simulink model "E5"  (Simulink 10.0)
settings: Solver=ode45  StartTime=0.0  StopTime=10.0  RelTol=1e-3  EnableMultiTasking=on
settings Model: Creator=tjohnson  LastModifiedBy=unknown
settings DataIOCC: LimitDataPoints=on
settings DebuggingCC: UnderspecifiedInitializationDetection=Simplified  MergeDetectMultiDrivingBlocksExec=error
settings GRTTargetCC: GeneratePreprocessorConditionals=Disable all  CombineOutputUpdateFcns=on  GRTInterface=off
settings ConfigComp: CovExternalEMLEnable=off

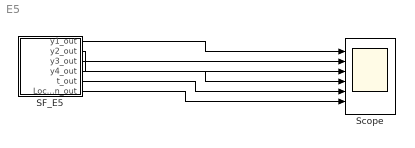
== system E5 ==
  SF_E5 : Stateflow chart  TreatAsAtomicUnit=on
  Scope : Scope  NumInputPorts=6
  wires:
  SF_E5/1(y1_out) -> Scope/1
  SF_E5/2(y2_out) -> Scope/2
  SF_E5/3(y3_out) -> Scope/3
  SF_E5/4(y4_out) -> Scope/4
  SF_E5/5(t_out) -> Scope/5
  SF_E5/6(Location_out) -> Scope/6

== stateflow chart SF_E5 ==
  settings: updateMethod=CONTINUOUS
  state E5
    du:
    y1_dot = -A * y1 - B * y1 * y3;
    y2_dot = A * y1 - M * C * y2 * y3;
    y3_dot = A * y1 - B * y1 * y3 - M * C * y2 * y3 + C * y4;
    y4_dot = B * y1 * y3 - C * y4;
    t_dot = 1.0;
    y1_out=y1;
    y2_out=y2;
    y3_out=y3;
    y4_out=y4;
    t_out=t;
    Location_out =1;
  (default) -> E5 : {t = 0.0; y1 = 0.00176; y2 = 0.0; y3 = 0.0; y4 = 0.0;}
  data: A constant double =7.89e-09; B constant double =11000000; C constant double =1130; M constant double =1000000; stop_time constant double =1000; y1 local double; y1_out output double; y2 local double; y2_out output double; y3 local double; y3_out output double; y4 local double; y4_out output double; t local double; t_out output double; Location_out output double
  data y1 settings: updateMethod=SF_CONTINUOUS_TIME_DATA
  data y2 settings: updateMethod=SF_CONTINUOUS_TIME_DATA
  data y3 settings: updateMethod=SF_CONTINUOUS_TIME_DATA
  data y4 settings: updateMethod=SF_CONTINUOUS_TIME_DATA
  data t settings: updateMethod=SF_CONTINUOUS_TIME_DATA
